simulink library "INT_Tra_TypeInfo"  (R2016b)
settings: Solver=VariableStepAuto  StartTime=0.0  StopTime=10.0  RelTol=1e-3
settings Model: Creator=Administrator  LastModifiedBy=Administrator

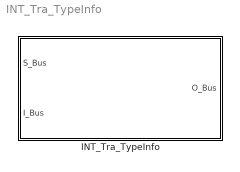
== system INT_Tra_TypeInfo ==
  INT_Tra_TypeInfo : Subsystem

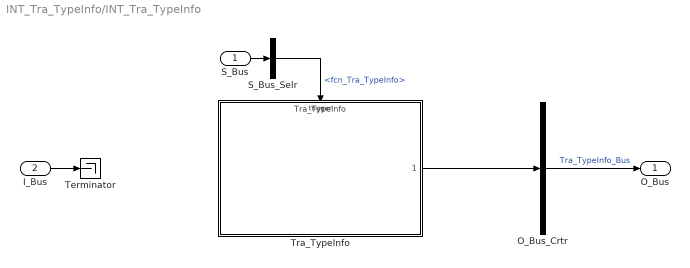
== system INT_Tra_TypeInfo/INT_Tra_TypeInfo ==
  S_Bus : Inport
  I_Bus : Inport  Port=2
  O_Bus_Crtr : BusCreator  Inputs=1
  S_Bus_Selr : BusSelector  OutputSignals=fcn_Tra_TypeInfo
  Terminator : Terminator
  Tra_TypeInfo : ModelReference  ModelNameDialog=Tra_TypeInfo  SimulationMode=Normal  ModelReferenceVersion=1.2  TriggerPortName=function  TriggerPortTriggerType=function-call  TriggerPortStatesWhenEnabling=held
  O_Bus : Outport
  wires:
  S_Bus_Selr/1 -> Tra_TypeInfo/Trigger  "<fcn_Tra_TypeInfo>"
  S_Bus/1 -> S_Bus_Selr/1
  I_Bus/1 -> Terminator/1
  O_Bus_Crtr/1 -> O_Bus/1  "Tra_TypeInfo_Bus"
  Tra_TypeInfo/1 -> O_Bus_Crtr/1
